simulink model "Model"  (R2024b)
settings: Solver=ode45  StartTime=0.0  StopTime=20  RelTol=1e-3
InitFcn:
  | Main
values from neighbouring files (symbols this model uses):
  A = [0, 1; 0, -10]    [Main.m]
  B = [0; 120]    [Main.m]
  C = [1, 0]    [Main.m]
  D = 0    [Main.m]
  Kw = 1 / (RiseTime / 5)    (= 33.3333333333)    [Main.m]
undefined symbols (not defined in the file or in its folder): KdRamp, KdStep, KiRamp, KiStep, KpRamp, KpStep, TlRamp, TlStep
settings Model: Creator=Banaan  LastModifiedBy=Banaan

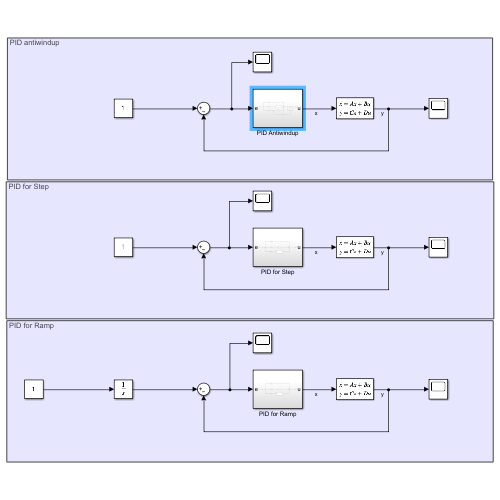
[thumbnail: Simulink's stored preview of the top-level diagram]
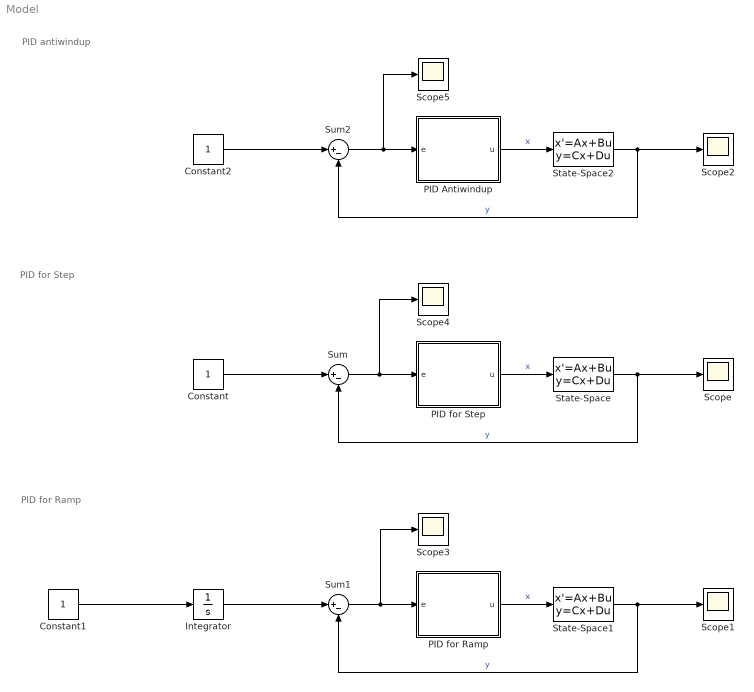
== system Model ==
  note: PID for Ramp
  note: PID for Step
  note: PID antiwindup
  Constant : Constant
  Constant1 : Constant
  Constant2 : Constant
  Integrator : Integrator
  PID Antiwindup : Subsystem
  PID for Ramp : Subsystem
  PID for Step : Subsystem
  Scope{,1..5} (6 alike) : Scope
  State-Space : StateSpace  A=A  B=B  C=C  D=D  InitialCondition=0
  State-Space1 : StateSpace  A=A  B=B  C=C  D=D  InitialCondition=0
  State-Space2 : StateSpace  A=A  B=B  C=C  D=D  InitialCondition=0
  Sum : Sum  Inputs=|+-
  Sum1 : Sum  Inputs=|+-
  Sum2 : Sum  Inputs=|+-
  wires:
  PID for Step/1(u) -> State-Space/1  "x"
  State-Space/1 -> Scope/1, Sum/2  "y"
  Constant/1 -> Sum/1
  Constant1/1 -> Integrator/1
  State-Space1/1 -> Scope1/1, Sum1/2  "y"
  Sum1/1 -> Scope3/1, PID for Ramp/1(e)
  PID for Ramp/1(u) -> State-Space1/1  "x"
  PID Antiwindup/1(u) -> State-Space2/1  "x"
  State-Space2/1 -> Sum2/2, Scope2/1  "y"
  Constant2/1 -> Sum2/1
  Integrator/1 -> Sum1/1
  Sum/1 -> Scope4/1, PID for Step/1(e)
  Sum2/1 -> Scope5/1, PID Antiwindup/1(e)

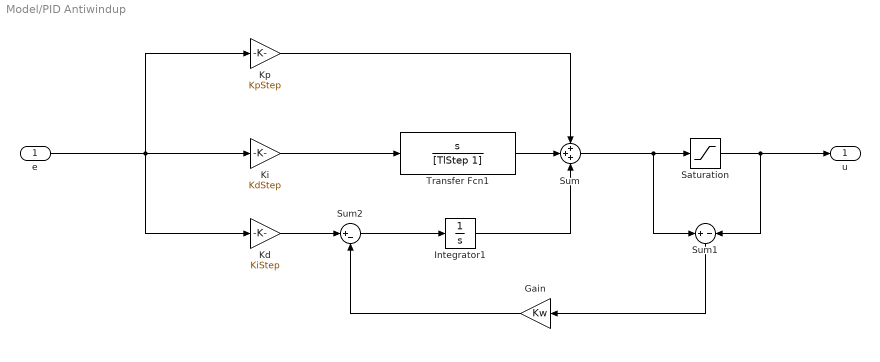
== system Model/PID Antiwindup ==
  e : Inport
  Gain : Gain  Gain=Kw
  Integrator1 : Integrator
  Kd : Gain  Gain=KiStep
  Ki : Gain  Gain=KdStep
  Kp : Gain  Gain=KpStep
  Saturation : Saturate  UpperLimit=10  LowerLimit=-10
  Sum : Sum  Inputs=+++
  Sum1 : Sum  Inputs=+|-
  Sum2 : Sum  Inputs=|+-
  Transfer Fcn1 : TransferFcn  Numerator=[1 0]  Denominator=[TlStep 1]
  u : Outport
  wires:
  Sum/1 -> Sum1/1, Saturation/1
  Transfer Fcn1/1 -> Sum/2
  Kp/1 -> Sum/1
  e/1 -> Ki/1, Kp/1, Kd/1
  Kd/1 -> Sum2/1
  Integrator1/1 -> Sum/3
  Ki/1 -> Transfer Fcn1/1
  Saturation/1 -> Sum1/2, u/1
  Sum2/1 -> Integrator1/1
  Gain/1 -> Sum2/2
  Sum1/1 -> Gain/1

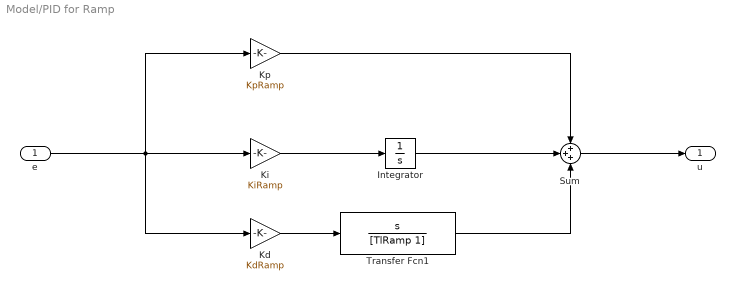
== system Model/PID for Ramp ==
  e : Inport
  Integrator : Integrator
  Kd : Gain  Gain=KdRamp
  Ki : Gain  Gain=KiRamp
  Kp : Gain  Gain=KpRamp
  Sum : Sum  Inputs=+++
  Transfer Fcn1 : TransferFcn  Numerator=[1 0]  Denominator=[TlRamp 1]
  u : Outport
  wires:
  Ki/1 -> Integrator/1
  Transfer Fcn1/1 -> Sum/3
  Kd/1 -> Transfer Fcn1/1
  e/1 -> Kd/1, Kp/1, Ki/1
  Kp/1 -> Sum/1
  Integrator/1 -> Sum/2
  Sum/1 -> u/1

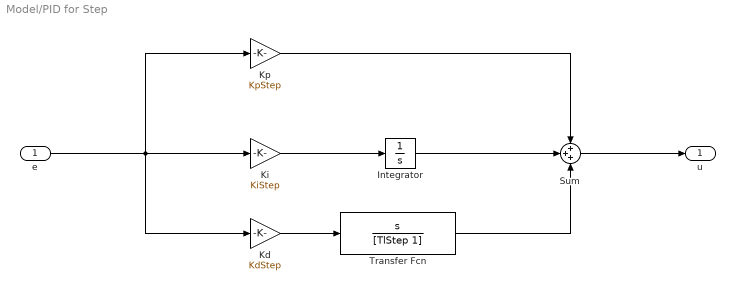
== system Model/PID for Step ==
  e : Inport
  Integrator : Integrator
  Kd : Gain  Gain=KdStep
  Ki : Gain  Gain=KiStep
  Kp : Gain  Gain=KpStep
  Sum : Sum  Inputs=+++
  Transfer Fcn : TransferFcn  Numerator=[1 0]  Denominator=[TlStep 1]
  u : Outport
  wires:
  Ki/1 -> Integrator/1
  Transfer Fcn/1 -> Sum/3
  Kd/1 -> Transfer Fcn/1
  e/1 -> Kd/1, Kp/1, Ki/1
  Kp/1 -> Sum/1
  Integrator/1 -> Sum/2
  Sum/1 -> u/1
